simulink model "IM_FluxController_Design"  (R2024b)
settings: Solver=VariableStepAuto  StartTime=0.0  StopTime=0.2  RelTol=1e-3
undefined symbols (not defined in the file): ctrl, en, im, lambda_Rd_ref, Ts
libraries: cstblocks x2
settings Model: Creator=overflow  LastModifiedBy=matth

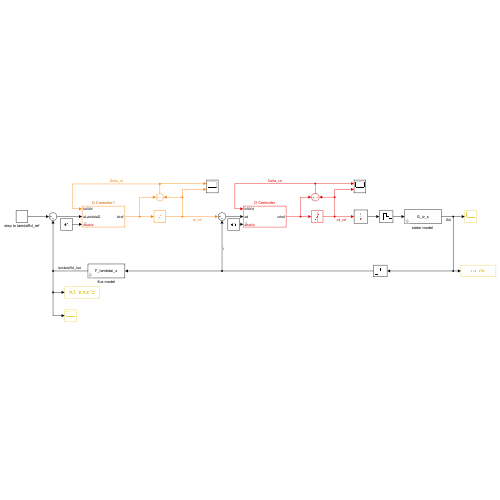
[thumbnail: Simulink's stored preview of the top-level diagram]
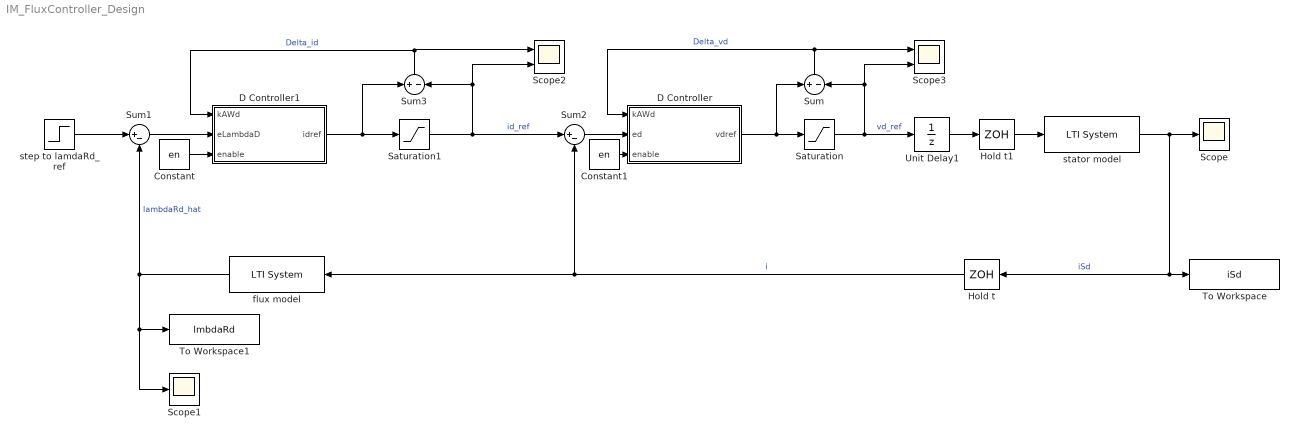
== system IM_FluxController_Design ==
  " Hold t" : ZeroOrderHold  SampleTime=Ts
  " Hold t1" : ZeroOrderHold  SampleTime=Ts
  Constant : Constant  Value=en
  Constant1 : Constant  Value=en
  D Controller : Subsystem  mask{Ts=ctrl.Ts, ctrl=ctrl.i}
      mask prompts: Ts "Sampling Time"; ctrl "Controller Struct"
  D Controller1 : Subsystem  mask{Ts=ctrl.Ts, ctrl=ctrl.lambda}
      mask prompts: Ts "Sampling Time"; ctrl "Controller Struct"
  Saturation : Saturate  UpperLimit=im.vSmax  LowerLimit=0  LinearizeAsGain=off
  Saturation1 : Saturate  UpperLimit=im.iSmax  LowerLimit=0
  Scope : Scope
  Scope1 : Scope
  Scope2 : Scope  NumInputPorts=2
  Scope3 : Scope  NumInputPorts=2
  Sum : Sum  Inputs=+|-
  Sum1 : Sum  Inputs=|+-
  Sum2 : Sum  Inputs=|+-
  Sum3 : Sum  Inputs=+|-
  To Workspace : ToWorkspace  VariableName=iSd  SaveFormat=Timeseries  SampleTime=-1
  To Workspace1 : ToWorkspace  VariableName=lmbdaRd  SaveFormat=Timeseries  SampleTime=-1
  Unit Delay1 : UnitDelay  SampleTime=Ts  HasFrameUpgradeWarning=on
  flux model : cstblocks/LTI System  sys=F_lambdai_z  IC=[0]  PadeOrder=0
  "stator model " : cstblocks/LTI System  sys=G_iv_s  IC=[0]  PadeOrder=0
  step to lamdaRd_ref : Step  Time=0  After=lambda_Rd_ref  SampleTime=0
  wires:
  Sum1/1 -> D Controller1/2(eLambdaD)
  flux model/1 -> Sum1/2, To Workspace1/1, Scope1/1  "lambdaRd_hat"
  " Hold t"/1 -> Sum2/2, flux model/1  "i"
  " Hold t1"/1 -> "stator model "/1
  "stator model "/1 -> Scope/1, " Hold t"/1, To Workspace/1  "iSd"
  Unit Delay1/1 -> " Hold t1"/1
  step to lamdaRd_ref/1 -> Sum1/1
  D Controller/1(vdref) -> Sum/1, Saturation/1
  Sum2/1 -> D Controller/2(ed)
  Saturation/1 -> Unit Delay1/1, Scope3/2, Sum/2  "vd_ref"
  Sum/1 -> Scope3/1, D Controller/1(kAWd)  "Delta_vd"
  Saturation1/1 -> Sum2/1, Scope2/2, Sum3/2  "id_ref"
  D Controller1/1(idref) -> Saturation1/1, Sum3/1
  Sum3/1 -> Scope2/1, D Controller1/1(kAWd)  "Delta_id"
  Constant/1 -> D Controller1/3(enable)
  Constant1/1 -> D Controller/3(enable)

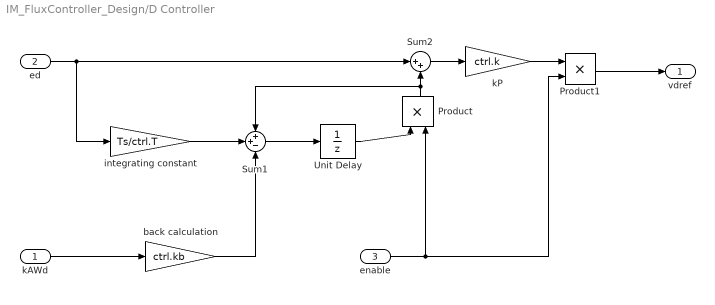
== system IM_FluxController_Design/D Controller ==
  kAWd : Inport
  ed : Inport  Port=2
  enable : Inport  Port=3
  Product : Product
  Product1 : Product
  Sum1 : Sum  Inputs=++-
  Sum2 : Sum  Inputs=|++
  Unit Delay : UnitDelay  SampleTime=-1  HasFrameUpgradeWarning=on
  back calculation : Gain  Gain=ctrl.kb
  integrating constant : Gain  Gain=Ts/ctrl.T
  kP : Gain  Gain=ctrl.k
  vdref : Outport
  wires:
  ed/1 -> integrating constant/1, Sum2/1
  Sum2/1 -> kP/1
  kAWd/1 -> back calculation/1
  Sum1/1 -> Unit Delay/1
  Unit Delay/1 -> Product/1
  Product/1 -> Sum1/1, Sum2/2
  kP/1 -> Product1/1
  Product1/1 -> vdref/1
  enable/1 -> Product1/2, Product/2
  integrating constant/1 -> Sum1/2
  back calculation/1 -> Sum1/3

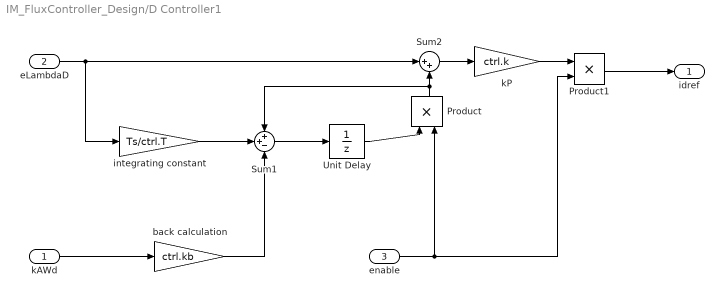
== system IM_FluxController_Design/D Controller1 ==
  kAWd : Inport
  eLambdaD : Inport  Port=2
  enable : Inport  Port=3
  Product : Product
  Product1 : Product
  Sum1 : Sum  Inputs=++-
  Sum2 : Sum  Inputs=|++
  Unit Delay : UnitDelay  SampleTime=-1  HasFrameUpgradeWarning=on
  back calculation : Gain  Gain=ctrl.kb
  integrating constant : Gain  Gain=Ts/ctrl.T
  kP : Gain  Gain=ctrl.k
  idref : Outport
  wires:
  eLambdaD/1 -> integrating constant/1, Sum2/1
  Sum2/1 -> kP/1
  kAWd/1 -> back calculation/1
  Sum1/1 -> Unit Delay/1
  Unit Delay/1 -> Product/1
  Product/1 -> Sum1/1, Sum2/2
  kP/1 -> Product1/1
  Product1/1 -> idref/1
  enable/1 -> Product1/2, Product/2
  integrating constant/1 -> Sum1/2
  back calculation/1 -> Sum1/3
